simulink model "IntegratedSim"  (R2018a)
settings: Solver=FixedStepDiscrete  StartTime=0.0  StopTime=10.0  FixedStep=Ts  RelTol=1e-3
values from neighbouring files (symbols this model uses):
  Ts = .01    (= 0.01)    [CubliConfig.m]
libraries: aerolibutil x5, vrlib x4, dspmtrx3 x1
settings Model: Creator=henry  LastModifiedBy=henry

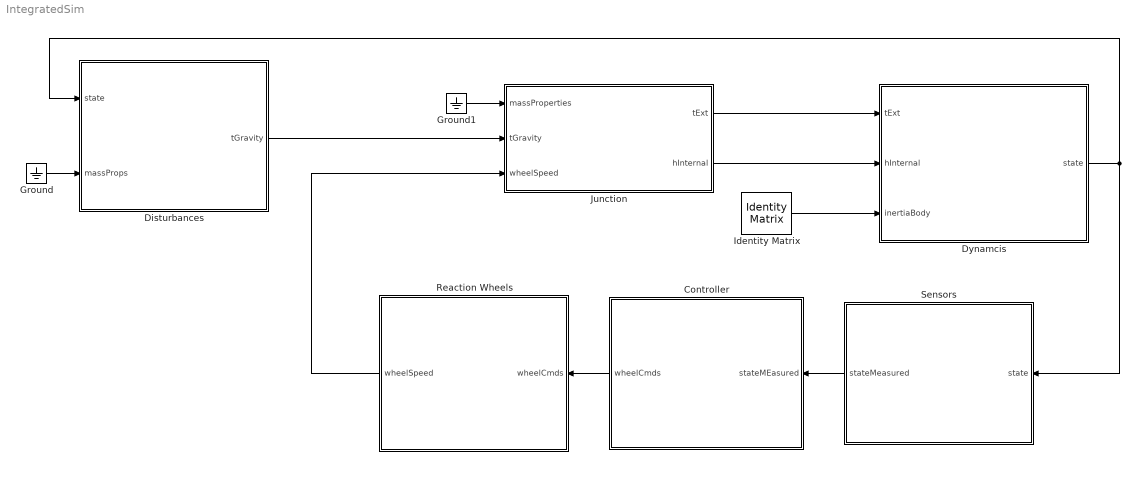
== system IntegratedSim ==
  Controller : Subsystem
  Disturbances : Subsystem
  Dynamcis : Subsystem
  Ground : Ground
  Ground1 : Ground
  Identity Matrix : dspmtrx3/Identity Matrix  Inherit=off  N=3  Ts=1  dataType=double  isSigned=on  wordLen=16  udDataType=sfix(16)  fracBitsMode=Best precision  numFracBits=15  OutDataTypeStr=double  LastOutDataTypeStr=double
      settings: SourceProductName=DSP System Toolbox
  Junction : Subsystem
  Reaction Wheels : Subsystem
  Sensors : Subsystem
  wires:
  Dynamcis/1(state) -> Disturbances/1(state), Sensors/1(state)
  Sensors/1(stateMeasured) -> Controller/1(stateMEasured)
  Controller/1(wheelCmds) -> Reaction Wheels/1(wheelCmds)
  Reaction Wheels/1(wheelSpeed) -> Junction/3(wheelSpeed)
  Disturbances/1(tGravity) -> Junction/2(tGravity)
  Junction/1(tExt) -> Dynamcis/1(tExt)
  Junction/2(hInternal) -> Dynamcis/2(hInternal)
  Identity Matrix/1 -> Dynamcis/3(inertiaBody)
  Ground/1 -> Disturbances/2(massProps)
  Ground1/1 -> Junction/1(massProperties)

== system IntegratedSim/Controller ==
  stateMEasured : Inport
  wheelCmds : Outport
  wires:
  stateMEasured/1 -> wheelCmds/1

== system IntegratedSim/Disturbances ==
  state : Inport
  massProps : Inport  Port=2
  Ground : Ground
  Terminator : Terminator
  Terminator1 : Terminator
  tGravity : Outport
  wires:
  state/1 -> Terminator/1
  massProps/1 -> Terminator1/1
  Ground/1 -> tGravity/1

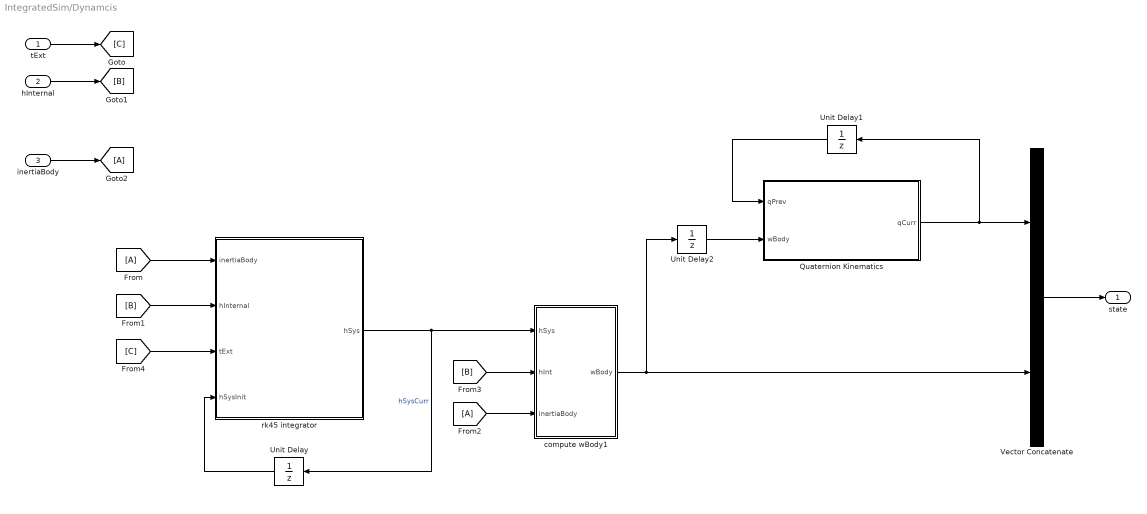
== system IntegratedSim/Dynamcis ==
  tExt : Inport
  hInternal : Inport  Port=2
  inertiaBody : Inport  Port=3
  Quaternion Kinematics : Subsystem
  Unit Delay : UnitDelay  InitialCondition=[1 1 1]  SampleTime=-1
  Unit Delay1 : UnitDelay  InitialCondition=[1 2 3 4]  SampleTime=-1
  Unit Delay2 : UnitDelay  InitialCondition=[1 1 1]  SampleTime=-1
  Vector Concatenate : Concatenate
  compute wBody1 : Subsystem
  rk45 integrator : Subsystem
  state : Outport
  wires:
  inertiaBody/1 -> [A]
  Unit Delay/1 -> rk45 integrator/4(hSysInit)
  Quaternion Kinematics/1(qCurr) -> Unit Delay1/1, Vector Concatenate/1
  Unit Delay1/1 -> Quaternion Kinematics/1(qPrev)
  [B] -> compute wBody1/2(hInt)
  rk45 integrator/1(hSys) -> Unit Delay/1, compute wBody1/1(hSys)  "hSysCurr"
  hInternal/1 -> [B]
  [B] -> rk45 integrator/2(hInternal)
  tExt/1 -> [C]
  Unit Delay2/1 -> Quaternion Kinematics/2(wBody)
  [C] -> rk45 integrator/3(tExt)
  [A] -> rk45 integrator/1(inertiaBody)
  Vector Concatenate/1 -> state/1
  [A] -> compute wBody1/3(inertiaBody)
  compute wBody1/1(wBody) -> Unit Delay2/1, Vector Concatenate/2

== system IntegratedSim/Junction ==
  massProperties : Inport
  tGravity : Inport  Port=2
  wheelSpeed : Inport  Port=3
  Terminator : Terminator
  tExt : Outport
  hInternal : Outport  Port=2
  wires:
  wheelSpeed/1 -> hInternal/1
  tGravity/1 -> tExt/1
  massProperties/1 -> Terminator/1

== system IntegratedSim/Reaction Wheels ==
  wheelCmds : Inport
  Ground : Ground
  Terminator : Terminator
  wheelSpeed : Outport
  wires:
  wheelCmds/1 -> Terminator/1
  Ground/1 -> wheelSpeed/1

== system IntegratedSim/Sensors ==
  state : Inport
  stateMeasured : Outport
  wires:
  state/1 -> stateMeasured/1

== system IntegratedSim/Dynamcis/Quaternion Kinematics ==
  qPrev : Inport
  wBody : Inport  Port=2
  Terminator : Terminator
  qCurr : Outport
  wires:
  qPrev/1 -> qCurr/1
  wBody/1 -> Terminator/1

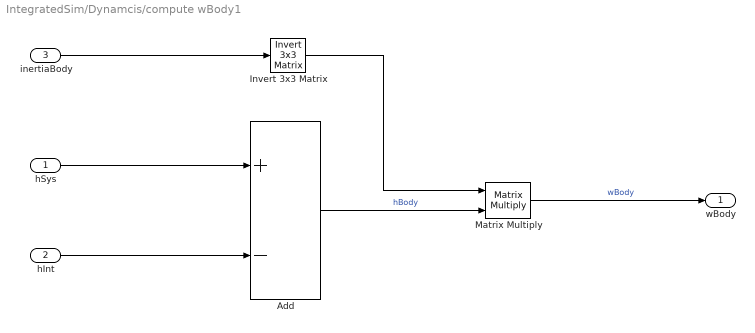
== system IntegratedSim/Dynamcis/compute wBody1 ==
  hSys : Inport
  hInt : Inport  Port=2
  inertiaBody : Inport  Port=3  OutDataTypeStr=double
  Add : Sum  Inputs=+-
  Invert 3x3 Matrix : aerolibutil/Invert  3x3 Matrix
  Matrix Multiply : Product  Multiplication=Matrix(*)
  wBody : Outport
  wires:
  Add/1 -> Matrix Multiply/2  "hBody"
  hInt/1 -> Add/2
  Invert 3x3 Matrix/1 -> Matrix Multiply/1
  Matrix Multiply/1 -> wBody/1  "wBody"
  hSys/1 -> Add/1
  inertiaBody/1 -> Invert 3x3 Matrix/1

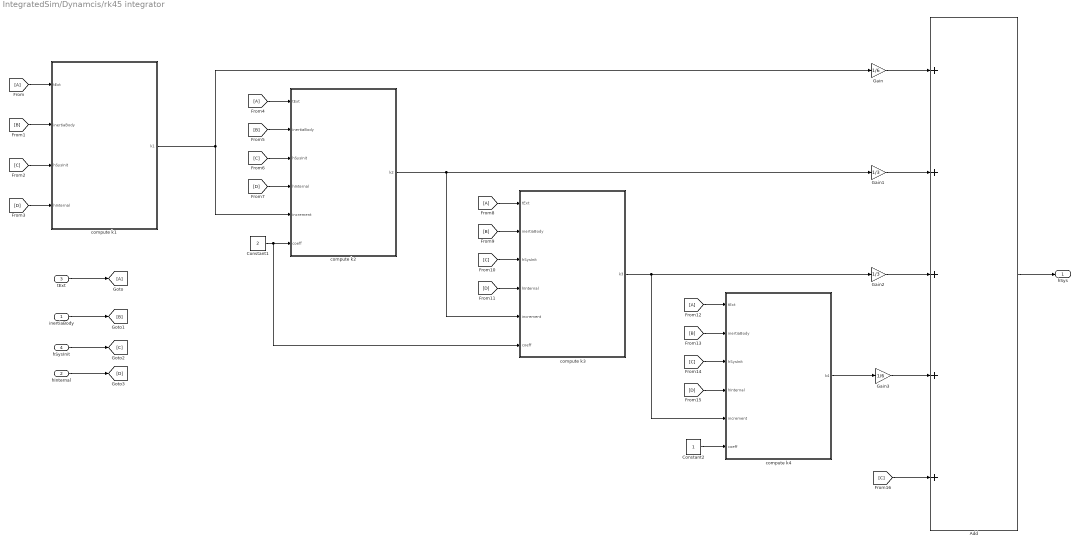
== system IntegratedSim/Dynamcis/rk45 integrator ==
  inertiaBody : Inport
  hInternal : Inport  Port=2
  tExt : Inport  Port=3
  hSysInit : Inport  Port=4
  Add : Sum  Inputs=+++++
  Constant1 : Constant  Value=2
  Constant2 : Constant
  Gain : Gain  Gain=1/6
  Gain1 : Gain  Gain=1/3
  Gain2 : Gain  Gain=1/3
  Gain3 : Gain  Gain=1/6
  compute k1 : Subsystem
  compute k2 : Subsystem
  compute k3 : Subsystem
  compute k4 : Subsystem
  hSys : Outport
  wires:
  [A] -> compute k1/1(tExt)
  tExt/1 -> [A]
  inertiaBody/1 -> [B]
  hSysInit/1 -> [C]
  hInternal/1 -> [D]
  [B] -> compute k1/2(inertiaBody)
  [C] -> compute k1/3(hSysInit)
  [D] -> compute k1/4(hInternal)
  [B] -> compute k2/2(inertiaBody)
  [D] -> compute k2/4(hInternal)
  [A] -> compute k2/1(tExt)
  [C] -> compute k2/3(hSysInit)
  [B] -> compute k3/2(inertiaBody)
  [D] -> compute k3/4(hInternal)
  [A] -> compute k3/1(tExt)
  [C] -> compute k3/3(hSysInit)
  [B] -> compute k4/2(inertiaBody)
  [D] -> compute k4/4(hInternal)
  [A] -> compute k4/1(tExt)
  [C] -> compute k4/3(hSysInit)
  compute k1/1(k1) -> Gain/1, compute k2/5(increment)
  compute k2/1(k2) -> compute k3/5(increment), Gain1/1
  compute k3/1(k3) -> compute k4/5(increment), Gain2/1
  Constant2/1 -> compute k4/6(coeff)
  Constant1/1 -> compute k3/6(coeff), compute k2/6(coeff)
  compute k4/1(k4) -> Gain3/1
  Gain/1 -> Add/1
  Gain1/1 -> Add/2
  Gain2/1 -> Add/3
  Gain3/1 -> Add/4
  [C] -> Add/5
  Add/1 -> hSys/1

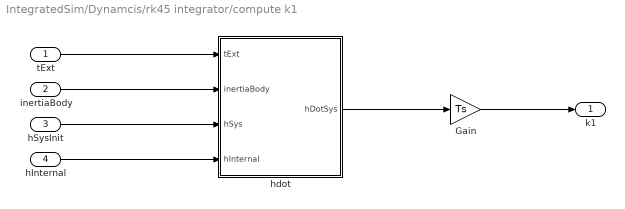
== system IntegratedSim/Dynamcis/rk45 integrator/compute k1 ==
  tExt : Inport
  inertiaBody : Inport  Port=2
  hSysInit : Inport  Port=3
  hInternal : Inport  Port=4
  Gain : Gain  Gain=Ts
  hdot : Subsystem
  k1 : Outport
  wires:
  hInternal/1 -> hdot/4(hInternal)
  inertiaBody/1 -> hdot/2(inertiaBody)
  tExt/1 -> hdot/1(tExt)
  hdot/1(hDotSys) -> Gain/1
  Gain/1 -> k1/1
  hSysInit/1 -> hdot/3(hSys)

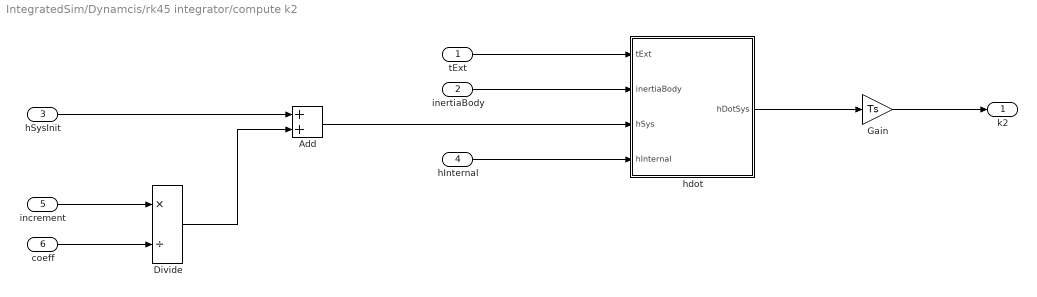
== system IntegratedSim/Dynamcis/rk45 integrator/compute k2 ==
  tExt : Inport
  inertiaBody : Inport  Port=2
  hSysInit : Inport  Port=3
  hInternal : Inport  Port=4
  increment : Inport  Port=5
  coeff : Inport  Port=6
  Add : Sum
  Divide : Product  Inputs=*/
  Gain : Gain  Gain=Ts
  hdot : Subsystem
  k2 : Outport
  wires:
  hInternal/1 -> hdot/4(hInternal)
  inertiaBody/1 -> hdot/2(inertiaBody)
  tExt/1 -> hdot/1(tExt)
  hSysInit/1 -> Add/1
  increment/1 -> Divide/1
  coeff/1 -> Divide/2
  Divide/1 -> Add/2
  Add/1 -> hdot/3(hSys)
  hdot/1(hDotSys) -> Gain/1
  Gain/1 -> k2/1

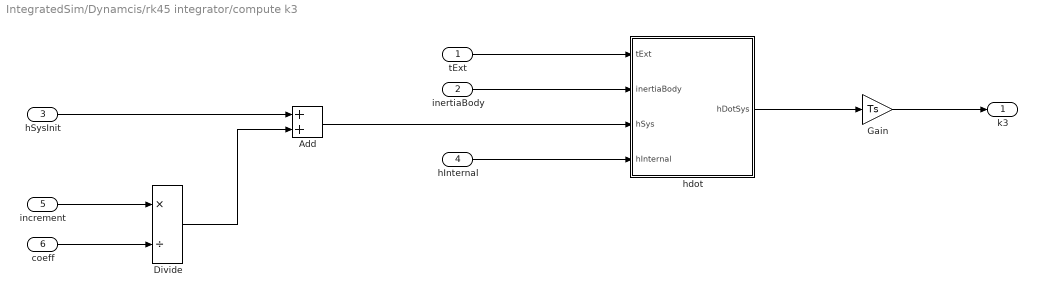
== system IntegratedSim/Dynamcis/rk45 integrator/compute k3 ==
  tExt : Inport
  inertiaBody : Inport  Port=2
  hSysInit : Inport  Port=3
  hInternal : Inport  Port=4
  increment : Inport  Port=5
  coeff : Inport  Port=6
  Add : Sum
  Divide : Product  Inputs=*/
  Gain : Gain  Gain=Ts
  hdot : Subsystem
  k3 : Outport
  wires:
  hInternal/1 -> hdot/4(hInternal)
  inertiaBody/1 -> hdot/2(inertiaBody)
  tExt/1 -> hdot/1(tExt)
  hSysInit/1 -> Add/1
  increment/1 -> Divide/1
  coeff/1 -> Divide/2
  Divide/1 -> Add/2
  Add/1 -> hdot/3(hSys)
  hdot/1(hDotSys) -> Gain/1
  Gain/1 -> k3/1

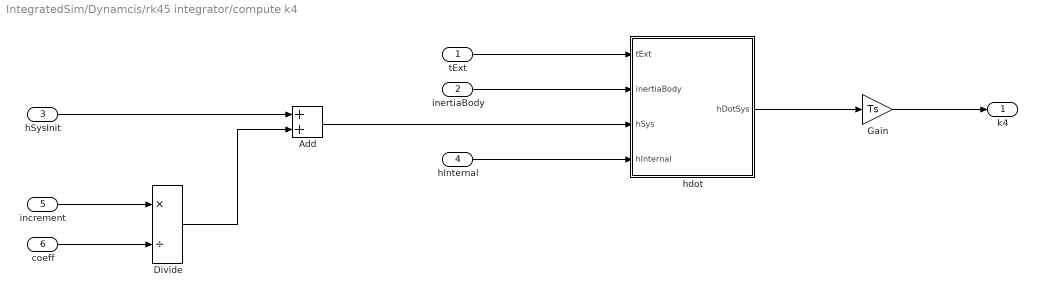
== system IntegratedSim/Dynamcis/rk45 integrator/compute k4 ==
  tExt : Inport
  inertiaBody : Inport  Port=2
  hSysInit : Inport  Port=3
  hInternal : Inport  Port=4
  increment : Inport  Port=5
  coeff : Inport  Port=6
  Add : Sum
  Divide : Product  Inputs=*/
  Gain : Gain  Gain=Ts
  hdot : Subsystem
  k4 : Outport
  wires:
  hInternal/1 -> hdot/4(hInternal)
  inertiaBody/1 -> hdot/2(inertiaBody)
  tExt/1 -> hdot/1(tExt)
  hSysInit/1 -> Add/1
  increment/1 -> Divide/1
  coeff/1 -> Divide/2
  Divide/1 -> Add/2
  Add/1 -> hdot/3(hSys)
  hdot/1(hDotSys) -> Gain/1
  Gain/1 -> k4/1

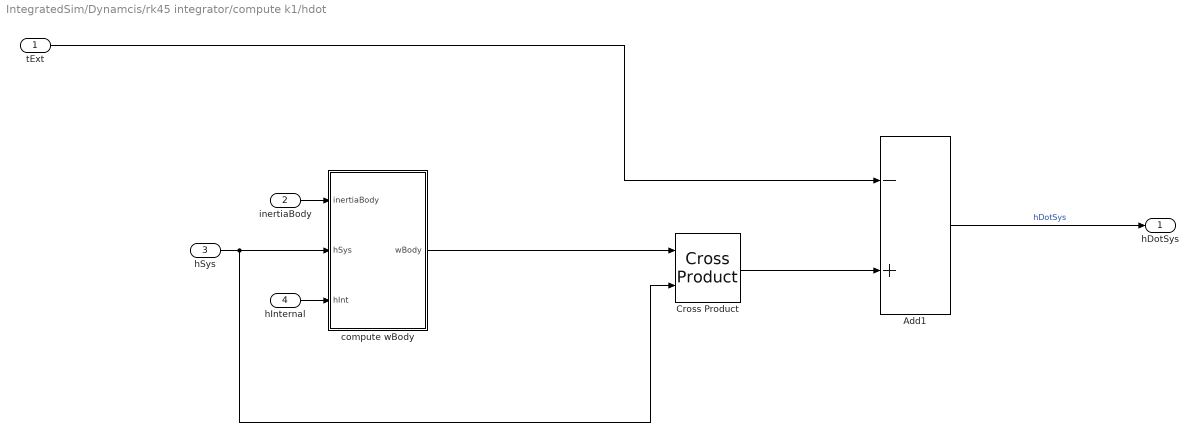
== system IntegratedSim/Dynamcis/rk45 integrator/compute k1/hdot ==
  tExt : Inport
  inertiaBody : Inport  Port=2
  hSys : Inport  Port=3
  hInternal : Inport  Port=4
  Add1 : Sum  Inputs=-+
  Cross Product : vrlib/Utilities/Cross Product
      settings: SourceProductBaseCode=VR
  compute wBody : Subsystem
  hDotSys : Outport
  wires:
  Add1/1 -> hDotSys/1  "hDotSys"
  tExt/1 -> Add1/1
  Cross Product/1 -> Add1/2
  inertiaBody/1 -> compute wBody/1(inertiaBody)
  hInternal/1 -> compute wBody/3(hInt)
  compute wBody/1(wBody) -> Cross Product/1
  hSys/1 -> Cross Product/2, compute wBody/2(hSys)

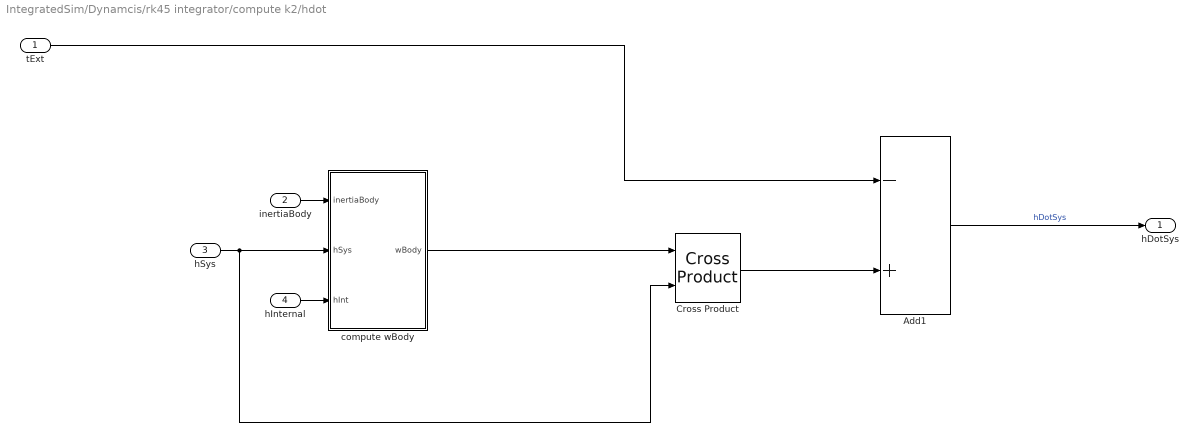
== system IntegratedSim/Dynamcis/rk45 integrator/compute k2/hdot ==
  tExt : Inport
  inertiaBody : Inport  Port=2
  hSys : Inport  Port=3
  hInternal : Inport  Port=4
  Add1 : Sum  Inputs=-+
  Cross Product : vrlib/Utilities/Cross Product
      settings: SourceProductBaseCode=VR
  compute wBody : Subsystem
  hDotSys : Outport
  wires:
  Add1/1 -> hDotSys/1  "hDotSys"
  tExt/1 -> Add1/1
  Cross Product/1 -> Add1/2
  inertiaBody/1 -> compute wBody/1(inertiaBody)
  hInternal/1 -> compute wBody/3(hInt)
  compute wBody/1(wBody) -> Cross Product/1
  hSys/1 -> Cross Product/2, compute wBody/2(hSys)

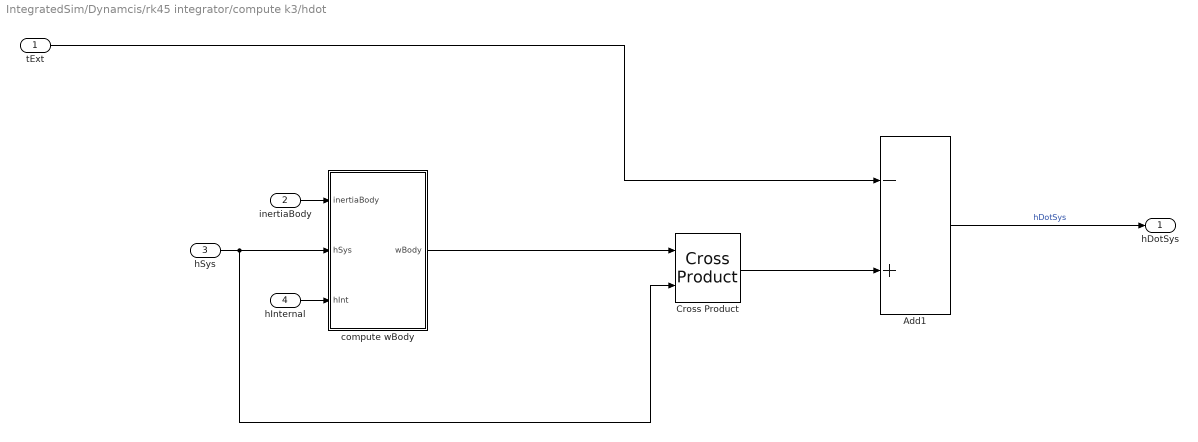
== system IntegratedSim/Dynamcis/rk45 integrator/compute k3/hdot ==
  tExt : Inport
  inertiaBody : Inport  Port=2
  hSys : Inport  Port=3
  hInternal : Inport  Port=4
  Add1 : Sum  Inputs=-+
  Cross Product : vrlib/Utilities/Cross Product
      settings: SourceProductBaseCode=VR
  compute wBody : Subsystem
  hDotSys : Outport
  wires:
  Add1/1 -> hDotSys/1  "hDotSys"
  tExt/1 -> Add1/1
  Cross Product/1 -> Add1/2
  inertiaBody/1 -> compute wBody/1(inertiaBody)
  hInternal/1 -> compute wBody/3(hInt)
  compute wBody/1(wBody) -> Cross Product/1
  hSys/1 -> Cross Product/2, compute wBody/2(hSys)

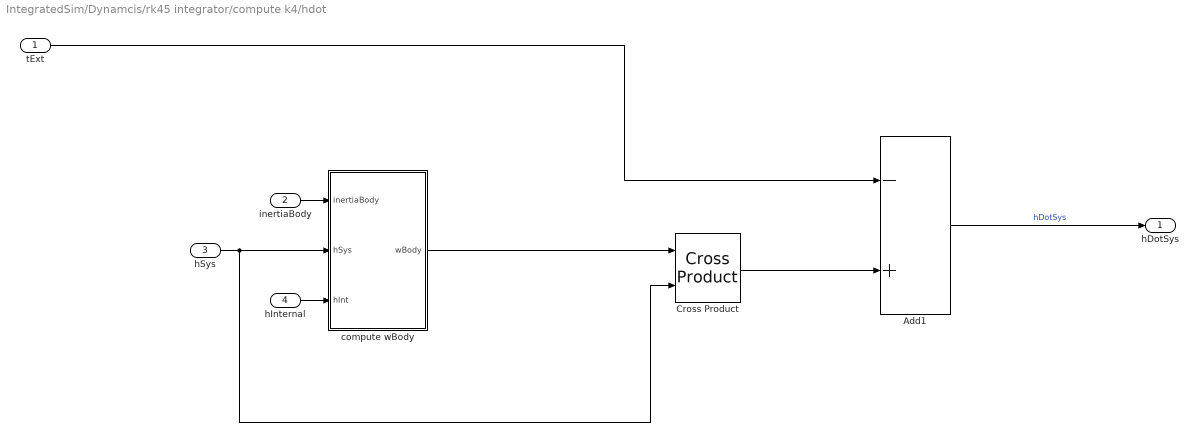
== system IntegratedSim/Dynamcis/rk45 integrator/compute k4/hdot ==
  tExt : Inport
  inertiaBody : Inport  Port=2
  hSys : Inport  Port=3
  hInternal : Inport  Port=4
  Add1 : Sum  Inputs=-+
  Cross Product : vrlib/Utilities/Cross Product
      settings: SourceProductBaseCode=VR
  compute wBody : Subsystem
  hDotSys : Outport
  wires:
  Add1/1 -> hDotSys/1  "hDotSys"
  tExt/1 -> Add1/1
  Cross Product/1 -> Add1/2
  inertiaBody/1 -> compute wBody/1(inertiaBody)
  hInternal/1 -> compute wBody/3(hInt)
  compute wBody/1(wBody) -> Cross Product/1
  hSys/1 -> Cross Product/2, compute wBody/2(hSys)

== system IntegratedSim/Dynamcis/rk45 integrator/compute k1/hdot/compute wBody ==
  inertiaBody : Inport
  hSys : Inport  Port=2
  hInt : Inport  Port=3
  Add : Sum  Inputs=+-
  Invert 3x3 Matrix : aerolibutil/Invert  3x3 Matrix
  Matrix Multiply : Product  Multiplication=Matrix(*)
  wBody : Outport
  wires:
  inertiaBody/1 -> Invert 3x3 Matrix/1
  hSys/1 -> Add/1
  Matrix Multiply/1 -> wBody/1  "wBody"
  Invert 3x3 Matrix/1 -> Matrix Multiply/1
  hInt/1 -> Add/2
  Add/1 -> Matrix Multiply/2  "hBody"

== system IntegratedSim/Dynamcis/rk45 integrator/compute k2/hdot/compute wBody ==
  inertiaBody : Inport
  hSys : Inport  Port=2
  hInt : Inport  Port=3
  Add : Sum  Inputs=+-
  Invert 3x3 Matrix : aerolibutil/Invert  3x3 Matrix
  Matrix Multiply : Product  Multiplication=Matrix(*)
  wBody : Outport
  wires:
  inertiaBody/1 -> Invert 3x3 Matrix/1
  hSys/1 -> Add/1
  Matrix Multiply/1 -> wBody/1  "wBody"
  Invert 3x3 Matrix/1 -> Matrix Multiply/1
  hInt/1 -> Add/2
  Add/1 -> Matrix Multiply/2  "hBody"

== system IntegratedSim/Dynamcis/rk45 integrator/compute k3/hdot/compute wBody ==
  inertiaBody : Inport
  hSys : Inport  Port=2
  hInt : Inport  Port=3
  Add : Sum  Inputs=+-
  Invert 3x3 Matrix : aerolibutil/Invert  3x3 Matrix
  Matrix Multiply : Product  Multiplication=Matrix(*)
  wBody : Outport
  wires:
  inertiaBody/1 -> Invert 3x3 Matrix/1
  hSys/1 -> Add/1
  Matrix Multiply/1 -> wBody/1  "wBody"
  Invert 3x3 Matrix/1 -> Matrix Multiply/1
  hInt/1 -> Add/2
  Add/1 -> Matrix Multiply/2  "hBody"

== system IntegratedSim/Dynamcis/rk45 integrator/compute k4/hdot/compute wBody ==
  inertiaBody : Inport
  hSys : Inport  Port=2
  hInt : Inport  Port=3
  Add : Sum  Inputs=+-
  Invert 3x3 Matrix : aerolibutil/Invert  3x3 Matrix
  Matrix Multiply : Product  Multiplication=Matrix(*)
  wBody : Outport
  wires:
  inertiaBody/1 -> Invert 3x3 Matrix/1
  hSys/1 -> Add/1
  Matrix Multiply/1 -> wBody/1  "wBody"
  Invert 3x3 Matrix/1 -> Matrix Multiply/1
  hInt/1 -> Add/2
  Add/1 -> Matrix Multiply/2  "hBody"
